simulink model "ssc_lead_acid_battery_mod1"  (R2017a)
settings: Solver=VariableStepAuto  StartTime=0.0  StopTime=36000  RelTol=1e-3  EnableMultiTasking=on
PreLoadFcn:
  | ssc_lead_acid_battery_ini
undefined symbols (not defined in the file): Kt, Kt_Temps, sigbuilder_block, theta_f, theta_init
libraries: fl_lib x15, nesl_utility x7, LeadAcidBattery_lib x6
CloseFcn:
  | try,close(h1_ssc_lead_acid_battery),end
  | clear h1_ssc_lead_acid_battery
  | 
  | clear simlog_ssc_lead_acid_battery
Description:
  | Lead-Acid Battery
  | 
  | Copyright 2012-2017 The MathWorks, Inc.
settings Model: Creator=MathWorks  LastModifiedBy=hlope
settings DataIOCC: LimitDataPoints=on  SaveFormat=Array
settings OptimizationCC: LifeSpan=inf
settings DebuggingCC: AllowSymbolicDim=off  SFUnexpectedBacktrackingDiag=warning  SFNoUnconditionalDefaultTransitionDiag=warning  SFExecutionAtInitializationDiag=none
settings HardwareCC: ProdBitPerPointer=32  ProdBitPerSizeT=32  ProdBitPerPtrDiffT=32  ProdLargestAtomicFloat=None  ProdIntDivRoundTo=Undefined  ProdEndianess=Unspecified  ProdWordSize=32  ProdHWDeviceType=32-bit Generic
settings ModelReferenceCC: PropagateSignalLabelsOutOfModel=off
settings GRTTargetCC: TargetLangStandard=C89/C90 (ANSI)  GeneratePreprocessorConditionals=Disable all
settings ConfigComp: CovMetricSettings=dw  CovHtmlReporting=on  CovSaveCumulativeToWorkspaceVar=on  CovSaveSingleToWorkspaceVar=on  CovExternalEMLEnable=off  CovSFcnEnable=off
settings SimscapeCC: SimscapeLogType=all  SimscapeLogSimulationStatistics=on  SimscapeLogName=simlog_ssc_lead_acid_battery  SimscapeLogDataHistory=10000

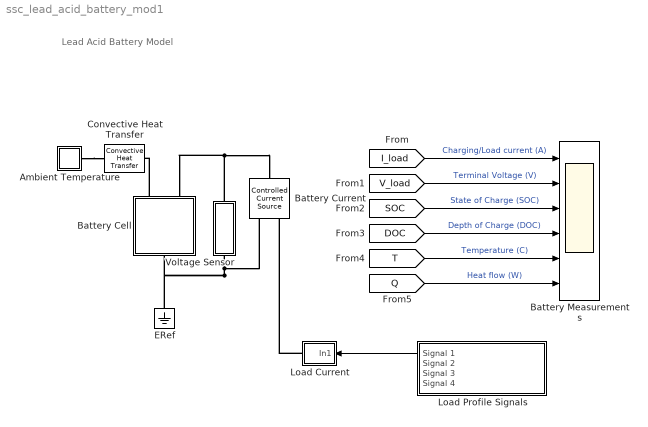
== system ssc_lead_acid_battery_mod1 ==
  note: Lead Acid Battery Model
  Ambient Temperature : Subsystem
      mask Display: disp('C')
  Battery Cell : Subsystem  Tag=PublishSubsystem
      mask Display:
      | % Battery icon
      | plot([0 0],[-1.5 -0.4])
      | plot([0 0 0.8 0.8],[0.2 0.9 0.9 1.5])
      | patch([-1 1 1 -1]*0.4,[1 1 -1 -1]*0.15-0.5,[0;0;0]);
      | patch([-1 1 1 -1]*0.9,[1 1 -1 -1]*0.15+0.1,[0;0;0]);
      | 
      | % Thermal port
      | plot([-1.2,-1.2],[0.5,0.9])
      | plot([-0.4,-0.4],[0.5,0.9])
      | plot([-0.8,-0.8],[0.9,1.5])
      | plot(0.35*cos(0:2*pi/50:2*pi)-0.8,0.15*sin(0:2*pi/50:2*pi)+0.85)
      | plot(0.35*cos(pi:2*pi/50:2*pi)-0.8,0.15*sin(pi:2*pi/50:2*pi)+0.55)
      | 
      | % Plot points to set plot range
      | color('white');plot(1.5,1.5);plot(-1.5,-1.5)
      | 
      | color('red')
      | port_label('LConn',1,'H')
      | port_label('LConn',2,'+')
      | port_label('RConn',1,'-')
  Battery Current : fl_lib/Electrical/Electrical Sources/Controlled Current Source
  Battery Measurements : Scope  NumInputPorts=6
  Convective Heat Transfer : fl_lib/Thermal/Thermal Elements/Convective Heat Transfer  area=Area m^2  heat_tr_coeff=Rtheta W/(m^2 * K)  Q_specify=off  Q_priority=High  Q=0 J/s  Q_nominal_specify=off  Q_nominal_unit=J/s  Q_nominal_value=1  T_specify=off  T_priority=High  T=0 K  T_nominal_specify=off  T_nominal_unit=K  T_nominal_value=1
  ERef : fl_lib/Electrical/Electrical Elements/Electrical Reference
  Load Current : Subsystem
  Load Profile Signals : Subsystem  Tag=STV Subsys  LoadFcn=sigbuilder_block('load');  StartFcn=sigbuilder_block('start');  StopFcn=sigbuilder_block('stop');  ClipboardFcn=sigbuilder_block('clipboard');  mask(Sigbuilder block){tuvar=[0:10]}
      mask help: Simulink:masks:SigbuilderBlock_MD
      mask init:
      | if ~strcmp(get_param(bdroot(gcbh),'SimulationStatus'),'stopped') tuvar = sigbuilder_block('maskInit'); end
      settings: CopyFcn=sigbuilder_block('copy');  DeleteFcn=sigbuilder_block('delete');  ModelCloseFcn=sigbuilder_block('modelClose');  PreSaveFcn=sigbuilder_block('preSave');  PauseFcn=sigbuilder_block('pause');  ContinueFcn=sigbuilder_block('continue');  NameChangeFcn=sigbuilder_block('namechange');  OpenFcn=sigbuilder_block('open',[571.8 30.6 574.8 516.6 ]);  CloseFcn=sigbuilder_block('close');
      mask Display: plot(0, 0, 100, 100,[2, 2, 32, 32, 2], [68, 8, 8, 68, 68],[32, 2], [38, 38], [32, 19, 2],[53, 60, 44], [32, 17, 17, 2],[16, 16, 31, 31]);txt = getActiveGroup(gcbh);text(2, 100, txt,'verticalAlignment', 'top');
  Voltage Sensor : Subsystem
      mask Display: disp('V_load')
  wires:
  [V_load] -> Battery Measurements/2  "Terminal Voltage (V)"
  [SOC] -> Battery Measurements/3  "State of Charge (SOC)"
  [DOC] -> Battery Measurements/4  "Depth of Charge (DOC)"
  [T] -> Battery Measurements/5  "Temperature (C)"
  [I_load] -> Battery Measurements/1  "Charging/Load current (A)"
  [Q] -> Battery Measurements/6  "Heat flow (W)"
  Load Profile Signals/1(Signal 1) -> Load Current/1(In1)
  connections:
  Voltage Sensor/RConn1 -- ERef/LConn1 -- Battery Cell/RConn1 -- Battery Current/RConn2
  Voltage Sensor/LConn1 -- Battery Cell/LConn2 -- Battery Current/LConn1
  Battery Cell/LConn1 -- Convective Heat Transfer/RConn1
  Ambient Temperature/RConn1 -- Convective Heat Transfer/LConn1
  Load Current/RConn1 -- Battery Current/RConn1

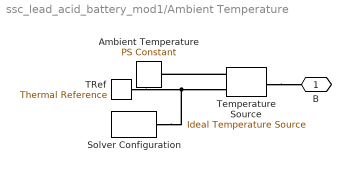
== system ssc_lead_acid_battery_mod1/Ambient Temperature ==
  Ambient Temperature : fl_lib/Physical Signals/Sources/PS Constant  constant=273+25
  Solver Configuration : nesl_utility/Solver Configuration  PhysicalDomain=network_engine_domain  SubClassName=solver  LeftPortType=input  RightPortType=generic  Accelerate=off  Tones=[]  Harmonics=[]  SimulateNoise=off  Profile=off  UseLocalSampling=off  EnableSwitchedLinearOptims=on  FrequencyDomain=off  UseCCode=off  RelTol=0.001  AbsTol=1e-06  MinStep=1e-09  ToWorkspace=off  RevertToSquareIcSolve=off  NumHomotopyIterations=100  PhasorMode=off  PhasorModeNumHarmonics=1  OverrideAbsTol=off  DoDC=off  ResidualTolerance=1e-9  UseLocalSolver=off  LocalSolverChoice=NE_BACKWARD_EULER_ADVANCER  LocalSolverSampleTime=1  DoFixedCost=off  MaxNonlinIter=3  MaxModeIter=2  LinearAlgebra=Sparse  DelaysMemoryBudget=1024  AutomaticFiltering=on  FilteringTimeConstant=0.001
  TRef : fl_lib/Thermal/Thermal Elements/Thermal Reference
  Temperature Source : fl_lib/Thermal/Thermal Sources/Ideal Temperature Source
      settings: SourceProductName=Simscape  SourceProductBaseCode=SS
  B : PMIOPort  Port=1  Side=Right
  connections:
  TRef/LConn1 -- Solver Configuration/RConn1 -- Temperature Source/RConn2
  Temperature Source/LConn1 -- B/RConn1
  Temperature Source/RConn1 -- Ambient Temperature/RConn1

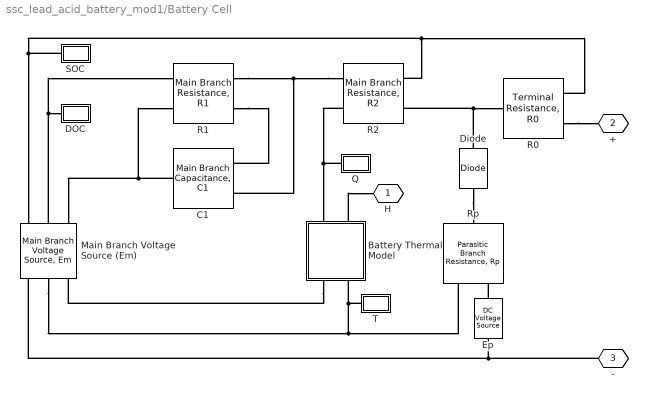
== system ssc_lead_acid_battery_mod1/Battery Cell ==
  " DOC " : Subsystem
  " SOC " : Subsystem
  Battery Thermal Model : Subsystem  Tag=PublishSubsystem
  C1 : LeadAcidBattery_lib/Main Branch Capacitance, C1  Tau1=Tau1 s  Cmin=1e-5 F
  Diode : fl_lib/Electrical/Electrical Elements/Diode  Vf=0.6 V  Ron=0.3 Ohm  Goff=1e-5 1/Ohm  i_specify=off  i_priority=High  i=0 A  i_nominal_specify=off  i_nominal_unit=A  i_nominal_value=1  v_specify=off  v_priority=High  v=0 V  v_nominal_specify=off  v_nominal_unit=V  v_nominal_value=1
  Ep : fl_lib/Electrical/Electrical Sources/DC Voltage Source  v0=Ep V
  Main Branch Voltage Source (Em) : LeadAcidBattery_lib/Main Branch Voltage Source, Em  Em0=Emo V  Ke=Ke V/K  Kc=Kc  C0=Costar s*A  Istar=Istar A  delta=delta  Tau1=Tau1 s  Qinit=Qe_init s*A
  Q : Subsystem
  R0 : LeadAcidBattery_lib/Terminal Resistance, R0  R00=Roo Ohm  A0=Ao
  R1 : LeadAcidBattery_lib/Main Branch Resistance, R1  R10=R10 Ohm  DOC_min=1e-006
  R2 : LeadAcidBattery_lib/Main Branch Resistance, R2  R20=R20 Ohm  A21=A21  A22=A22  Istar=Istar A
  Rp : LeadAcidBattery_lib/Parasitic Branch Resistance, Rp  Gp0=Gpo 1/Ohm  Vp0=Vpo V  Ap=Ap  Tf=theta_f degC
  T : Subsystem
  H : PMIOPort  Tag=PMCPort  Port=1  Side=Left
  + : PMIOPort  Tag=PMCPort  Port=2  Side=Left
  - : PMIOPort  Tag=PMCPort  Port=3  Side=Right
  connections:
  Battery Thermal Model/RConn2 -- T/LConn1 -- Rp/RConn1 -- Main Branch Voltage Source (Em)/RConn2
  R0/LConn2 -- +/RConn1
  " DOC "/LConn1 -- R1/RConn1 -- Main Branch Voltage Source (Em)/LConn2
  C1/RConn1 -- R1/RConn2 -- Main Branch Voltage Source (Em)/LConn3
  R2/RConn1 -- C1/LConn2 -- R1/LConn1
  R1/LConn2 -- C1/LConn1
  R0/LConn1 -- " SOC "/LConn1 -- Main Branch Voltage Source (Em)/LConn1 -- R2/LConn1
  Battery Thermal Model/LConn2 -- H/RConn1
  Ep/LConn1 -- Rp/RConn2
  Diode/RConn1 -- Rp/LConn1
  Battery Thermal Model/RConn1 -- Main Branch Voltage Source (Em)/RConn3
  Ep/RConn1 -- Main Branch Voltage Source (Em)/RConn1 -- -/RConn1
  R2/RConn2 -- Q/LConn1 -- Battery Thermal Model/LConn1
  R2/LConn2 -- R0/RConn1 -- Diode/LConn1

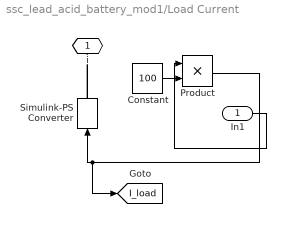
== system ssc_lead_acid_battery_mod1/Load Current ==
  In1 : Inport
  Constant : Constant  Value=100
  Product : Product
  Simulink-PS Converter : nesl_utility/Simulink-PS Converter  PhysicalDomain=network_engine_domain  SubClassName=ps_input  LeftPortType=input  RightPortType=output  PseudoPeriodic=off  Frequencies=[]  NoiseDistribution=none  NoiseParameters=[]  Unit=A  AffineConversion=off  FilteringAndDerivatives=zero  SimscapeFilterOrder=1  InputFilterTimeConstant=.001  UdotUserProvided=0
  i : PMIOPort  Port=1  Side=Right
  tag scope: I_load=global
  wires:
  Constant/1 -> Product/2
  In1/1 -> Product/1
  Product/1 -> [I_load], Simulink-PS Converter/1
  connections:
  Simulink-PS Converter/RConn1 -- i/RConn1

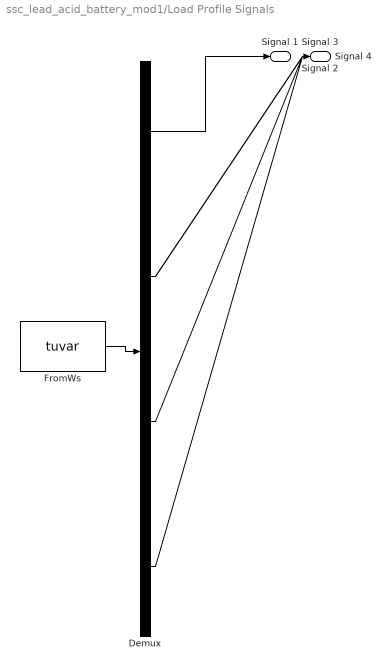
== system ssc_lead_acid_battery_mod1/Load Profile Signals ==
  Demux : Demux  Tag=STV Demux
  FromWs : FromWorkspace  Tag=STV FromWs  VariableName=tuvar  SampleTime=0
      SigBuilderData=|
      | common.afterFinalStr = 'Extrapolate'
      | common.sampleTime = 0
      | dataSet.timeRange = [0 3600]
      | dataSet.name = 'Group 1'
      | sbobj.Groups.Name = 'Group 1'
      | sbobj.Groups.Signals(1).Name = 'Signal 1'
      | sbobj.Groups.Signals(1).XData = [0 500 500 990 990 2640 2640 3500 3500 3600]
      | sbobj.Groups.Signals(1).YData = [0 0 1 1 0 -0.0011877394636 0.49 0.49 0 0]
      | sbobj.Groups.Signals(2).Name = 'Signal 2'
      | sbobj.Groups.Signals(2).XData = [0 300 300 700 700 800 800 1000 1000 1100 1100 1500 1500 1600 1600 1700 1700 1800 1800 1900 1900 2000 2000 2100 2100 2200 2200 2400 2400 2600 2600 2800 2800 3000 3000 3300 3300 3400 3400 3600 3600]
      | sbobj.Groups.Signals(2).YData = [1 1 0 0 1 1 0 0 1 1 0 0 1 1 0 0 1 1 0 0 1 1 0 0 1 1 0 0 1 1 0 0 1 1 0 0 1 1 0 0 1]
      | sbobj.Groups.Signals(3).Name = 'Signal 3'
      | sbobj.Groups.Signals(3).XData = [0 0.5 0.5 1 1 1.5 1.5 2 2 2.5 2.5 3 3 3.5 3.5 4 4 4.5 4.5 5 5 5.5 5.5 6 6 6.5 6.5 7 7 7.5 7.5 8 8 8.5 8.5 9 9 9.5 9.5 3600]
      | sbobj.Groups.Signals(3).YData = [2 2 0 0 2 2 0 0 2 2 0 0 2 2 0 0 2 2 0 0 2 2 0 0 2 2 0 0 2 2 0 0 2 2 0 0 2 2 0 0]
      | sbobj.Groups.Signals(4).Name = 'Signal 4'
      | sbobj.Groups.Signals(4).XData = [0 3600]
      | sbobj.Groups.Signals(4).YData = [0 0]
      | sbobj.Groups.TimeRange = [0 3600]
  Signal 1 : Outport  Tag=STV Outport
  Signal 2 : Outport  Tag=STV Outport  Port=2
  Signal 3 : Outport  Tag=STV Outport  Port=3
  Signal 4 : Outport  Tag=STV Outport  Port=4
  wires:
  Demux/1 -> Signal 1/1
  FromWs/1 -> Demux/1
  Demux/2 -> Signal 2/1
  Demux/3 -> Signal 3/1
  Demux/4 -> Signal 4/1

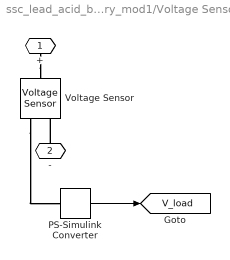
== system ssc_lead_acid_battery_mod1/Voltage Sensor ==
  PS-Simulink Converter : nesl_utility/PS-Simulink Converter  PhysicalDomain=network_engine_domain  SubClassName=ps_output  LeftPortType=input  RightPortType=output  PseudoPeriodic=off  Frequencies=[]  Unit=V  AffineConversion=off
  Voltage Sensor : fl_lib/Electrical/Electrical Sensors/Voltage Sensor
  + : PMIOPort  Port=1  Side=Left
  - : PMIOPort  Port=2  Side=Right
  tag scope: V_load=global
  wires:
  PS-Simulink Converter/1 -> [V_load]
  connections:
  Voltage Sensor/RConn1 -- PS-Simulink Converter/LConn1
  +/RConn1 -- Voltage Sensor/LConn1
  -/RConn1 -- Voltage Sensor/RConn2

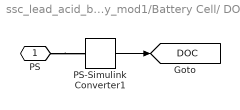
== system ssc_lead_acid_battery_mod1/Battery Cell/ DOC  ==
  PS-Simulink Converter1 : nesl_utility/PS-Simulink Converter  PhysicalDomain=network_engine_domain  SubClassName=ps_output  LeftPortType=input  RightPortType=output  PseudoPeriodic=off  Frequencies=[]  Unit=1  AffineConversion=off
  PS : PMIOPort  Port=1  Side=Left
  tag scope: DOC=global
  wires:
  PS-Simulink Converter1/1 -> [DOC]
  connections:
  PS/RConn1 -- PS-Simulink Converter1/LConn1

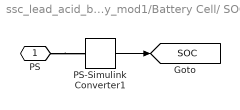
== system ssc_lead_acid_battery_mod1/Battery Cell/ SOC  ==
  PS-Simulink Converter1 : nesl_utility/PS-Simulink Converter  PhysicalDomain=network_engine_domain  SubClassName=ps_output  LeftPortType=input  RightPortType=output  PseudoPeriodic=off  Frequencies=[]  Unit=1  AffineConversion=off
  PS : PMIOPort  Port=1  Side=Left
  tag scope: SOC=global
  wires:
  PS-Simulink Converter1/1 -> [SOC]
  connections:
  PS/RConn1 -- PS-Simulink Converter1/LConn1

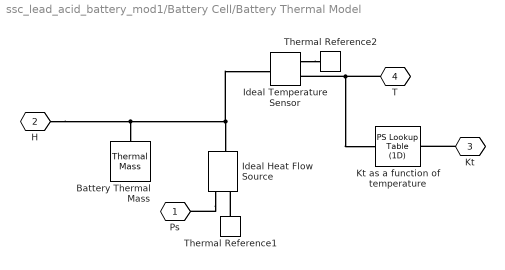
== system ssc_lead_acid_battery_mod1/Battery Cell/Battery Thermal Model ==
  Battery Thermal Mass : fl_lib/Thermal/Thermal Elements/Thermal Mass  mass=1 kg  sp_heat=Ctheta J/kg/K  T_specify=on  T_priority=High  T=theta_init degC  T_nominal_specify=off  T_nominal_unit=K  T_nominal_value=1  Q_specify=off  Q_priority=High  Q=0 J/s  Q_nominal_specify=off  Q_nominal_unit=J/s  Q_nominal_value=1
  Ideal Temperature Sensor : fl_lib/Thermal/Thermal Sensors/Ideal Temperature Sensor
      settings: SourceProductName=Simscape  SourceProductBaseCode=SS
  Ideal Heat Flow Source : fl_lib/Thermal/Thermal Sources/Ideal Heat Flow Source
      settings: SourceProductName=Simscape  SourceProductBaseCode=SS
  Kt as a function of temperature : fl_lib/Physical Signals/Lookup Tables/PS Lookup Table (1D)  x=[theta_f, Kt_Temps]+273  f=[0 Kt]  interp_method=1  extrap_method=1
      settings: SourceProductName=Simscape  SourceProductBaseCode=SS
  Thermal Reference1 : fl_lib/Thermal/Thermal Elements/Thermal Reference
  Thermal Reference2 : fl_lib/Thermal/Thermal Elements/Thermal Reference
  Ps : PMIOPort  Tag=PMCPort  Port=1  Side=Left
  H : PMIOPort  Tag=PMCPort  Port=2  Side=Left
  Kt : PMIOPort  Tag=PMCPort  Port=3  Side=Right
  T : PMIOPort  Tag=PMCPort  Port=4  Side=Right
  connections:
  Ideal Temperature Sensor/RConn1 -- Thermal Reference2/LConn1
  Ideal Temperature Sensor/RConn2 -- Kt as a function of temperature/LConn1 -- T/RConn1
  Thermal Reference1/LConn1 -- Ideal Heat Flow Source/RConn2
  H/RConn1 -- Ideal Temperature Sensor/LConn1 -- Ideal Heat Flow Source/LConn1 -- Battery Thermal Mass/LConn1
  Kt/RConn1 -- Kt as a function of temperature/RConn1
  Ideal Heat Flow Source/RConn1 -- Ps/RConn1

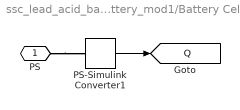
== system ssc_lead_acid_battery_mod1/Battery Cell/Q ==
  PS-Simulink Converter1 : nesl_utility/PS-Simulink Converter  PhysicalDomain=network_engine_domain  SubClassName=ps_output  LeftPortType=input  RightPortType=output  PseudoPeriodic=off  Frequencies=[]  Unit=W  AffineConversion=on
  PS : PMIOPort  Port=1  Side=Left
  tag scope: Q=global
  wires:
  PS-Simulink Converter1/1 -> [Q]
  connections:
  PS/RConn1 -- PS-Simulink Converter1/LConn1

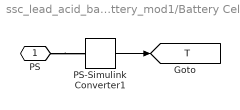
== system ssc_lead_acid_battery_mod1/Battery Cell/T ==
  PS-Simulink Converter1 : nesl_utility/PS-Simulink Converter  PhysicalDomain=network_engine_domain  SubClassName=ps_output  LeftPortType=input  RightPortType=output  PseudoPeriodic=off  Frequencies=[]  Unit=degC  AffineConversion=on
  PS : PMIOPort  Port=1  Side=Left
  tag scope: T=global
  wires:
  PS-Simulink Converter1/1 -> [T]
  connections:
  PS/RConn1 -- PS-Simulink Converter1/LConn1
